simulink model "WheelSpeed"  (R2020b)
settings: Solver=VariableStepAuto  StartTime=0.0  StopTime=10.0  RelTol=1e-3
PreLoadFcn:
  | abs_data;
model workspace (MAT data in the model file):
  I = 5
  TB = 0.01
  kf = 1
undefined symbols (not defined in the file): Rr
settings Model: OrderedModelArguments=off  Creator=ADMIN  LastModifiedBy=ADMIN
settings DataIOCC: SaveOutput=off  SaveTime=off

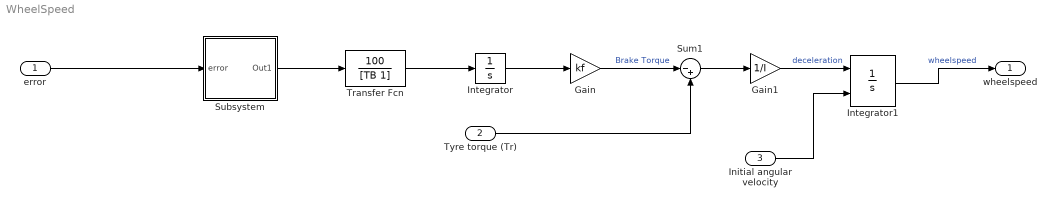
== system WheelSpeed ==
  error : Inport  OutDataTypeStr=double  PortDimensions=1  SampleTime=0
  Tyre torque (Tr) : Inport  Port=2  OutDataTypeStr=double  PortDimensions=1  SampleTime=0
  Initial angular velocity : Inport  Port=3
  Gain : Gain  Gain=kf
  Gain1 : Gain  Gain=1/I
  Integrator : Integrator  LimitOutput=on  UpperSaturationLimit=1000  LowerSaturationLimit=0
  Integrator1 : Integrator  InitialConditionSource=external  InitialCondition=88/Rr  LimitOutput=on  UpperSaturationLimit=1000  LowerSaturationLimit=0
  Subsystem : Subsystem
  Sum1 : Sum  Inputs=|-+
  Transfer Fcn : TransferFcn  Numerator=[100]  Denominator=[TB 1]
  wheelspeed : Outport  OutDataTypeStr=double  PortDimensions=1  SampleTime=0
  wires:
  Sum1/1 -> Gain1/1
  error/1 -> Subsystem/1(error)
  Transfer Fcn/1 -> Integrator/1
  Gain1/1 -> Integrator1/1  "deceleration"
  Integrator1/1 -> wheelspeed/1  "wheelspeed"
  Integrator/1 -> Gain/1
  Gain/1 -> Sum1/1  "Brake Torque"
  Tyre torque (Tr)/1 -> Sum1/2
  Subsystem/1(Out1) -> Transfer Fcn/1
  Initial angular velocity/1 -> Integrator1/2

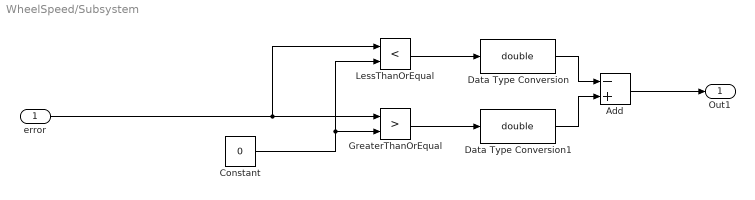
== system WheelSpeed/Subsystem ==
  error : Inport
  Add : Sum  Inputs=-+
  Constant : Constant  Value=0
  Data Type Conversion : DataTypeConversion  OutDataTypeStr=double
  Data Type Conversion1 : DataTypeConversion  OutDataTypeStr=double
  GreaterThanOrEqual : RelationalOperator  Operator=>  OutDataTypeStr=boolean  RndMeth=Simplest
  LessThanOrEqual : RelationalOperator  Operator=<  OutDataTypeStr=boolean  RndMeth=Simplest
  Out1 : Outport
  wires:
  GreaterThanOrEqual/1 -> Data Type Conversion1/1
  LessThanOrEqual/1 -> Data Type Conversion/1
  Data Type Conversion1/1 -> Add/2
  Add/1 -> Out1/1
  Constant/1 -> GreaterThanOrEqual/2, LessThanOrEqual/2
  Data Type Conversion/1 -> Add/1
  error/1 -> GreaterThanOrEqual/1, LessThanOrEqual/1
